simulink subsystem "Communication_Simulator"  (R2024a)
settings: Solver=VariableStepAuto  StartTime=0.0  StopTime=10.0  RelTol=1e-3
undefined symbols (not defined in the file): paramRFSatLink, QAM, rfSatSourceSamplesPerSymbol, rfSatSourceSampleTime
libraries: commrflib2 x24, dspsigops x12, commrfcorlib x8, commfilt2 x8, commdigbbndam3 x8, dspsolvers x8, simulink x8, commrandsrc3 x4, commsink2 x4, commdemoslib x4, impairlib x4, commsync2 x4
(part 3 of 3)

== system Communication_Simulator/TT&C Communication/Ground Segment/Downlink/Nonlinearity/Digital Pre-Distortion ==
  In1 : Inport
  In2 : Inport  Port=2
  Distortion compensation : Subsystem
  Parameter Estimation : Subsystem
  Out1 : Outport  VectorParamsAs1DForOutWhenUnconnected=off
  wires:
  In1/1 -> Distortion compensation/3(In), Parameter Estimation/1(DUT Input)
  Parameter Estimation/1(c) -> Distortion compensation/1(c)
  Parameter Estimation/2(d) -> Distortion compensation/2(d)
  Distortion compensation/1(Pre-distorted Signal) -> Out1/1
  In2/1 -> Parameter Estimation/2(DUT Output)

== system Communication_Simulator/TT&C Communication/Ground Segment/Ground Station/Nonlinearity1/Digital Pre-Distortion ==
  In1 : Inport
  In2 : Inport  Port=2
  Distortion compensation : Subsystem
  Parameter Estimation : Subsystem
  Out1 : Outport  VectorParamsAs1DForOutWhenUnconnected=off
  wires:
  In1/1 -> Distortion compensation/3(In), Parameter Estimation/1(DUT Input)
  Parameter Estimation/1(c) -> Distortion compensation/1(c)
  Parameter Estimation/2(d) -> Distortion compensation/2(d)
  Distortion compensation/1(Pre-distorted Signal) -> Out1/1
  In2/1 -> Parameter Estimation/2(DUT Output)

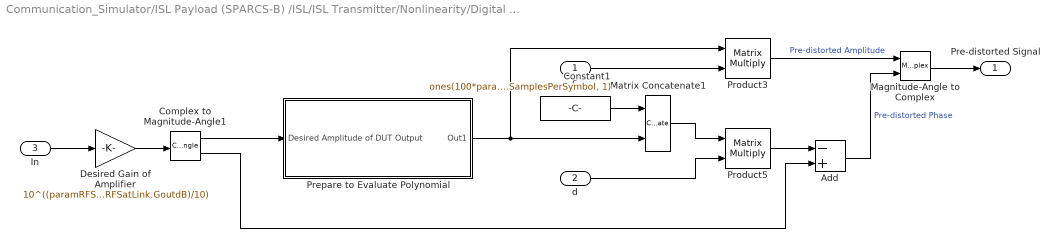
== system Communication_Simulator/ISL Payload (SPARCS-B) /ISL/ISL Transmitter/Nonlinearity/Digital Pre-Distortion/Distortion compensation ==
  c : Inport
  d : Inport  Port=2
  In : Inport  Port=3
  Add : Sum  Inputs=-+
  Complex to Magnitude-Angle1 : ComplexToMagnitudeAngle
  Constant1 : Constant  Value=ones(100*paramRFSatLink.SamplesPerSymbol, 1)
  Desired Gain of Amplifier : Gain  Gain=10^((paramRFSatLink.GindB + paramRFSatLink.GoutdB)/10)
  Magnitude-Angle to Complex : MagnitudeAngleToComplex
  Matrix Concatenate1 : Concatenate  Mode=Multidimensional array  ConcatenateDimension=2
  Prepare to Evaluate Polynomial : Subsystem
  Product3 : Product  Multiplication=Matrix(*)  RndMeth=Zero
  Product5 : Product  Multiplication=Matrix(*)  RndMeth=Zero
  Pre-distorted Signal : Outport  VectorParamsAs1DForOutWhenUnconnected=off
  wires:
  Desired Gain of Amplifier/1 -> Complex to Magnitude-Angle1/1
  c/1 -> Product3/2
  Add/1 -> Magnitude-Angle to Complex/2  "Pre-distorted Phase"
  Product5/1 -> Add/1
  Product3/1 -> Magnitude-Angle to Complex/1  "Pre-distorted Amplitude"
  d/1 -> Product5/2
  In/1 -> Desired Gain of Amplifier/1
  Magnitude-Angle to Complex/1 -> Pre-distorted Signal/1
  Complex to Magnitude-Angle1/2 -> Add/2
  Complex to Magnitude-Angle1/1 -> Prepare to Evaluate Polynomial/1(Desired Amplitude of DUT Output)
  Matrix Concatenate1/1 -> Product5/1
  Prepare to Evaluate Polynomial/1(Out1) -> Matrix Concatenate1/2, Product3/1
  Constant1/1 -> Matrix Concatenate1/1

== system Communication_Simulator/ISL Payload (SPARCS-B) /ISL/ISL Transmitter/Nonlinearity/Digital Pre-Distortion/Parameter Estimation ==
  DUT Input : Inport
  DUT Output : Inport  Port=2
  Complex to Magnitude-Angle : ComplexToMagnitudeAngle
  Complex to Magnitude-Angle1 : ComplexToMagnitudeAngle
  Polynomial Approximation : Subsystem
  c : Outport  VectorParamsAs1DForOutWhenUnconnected=off
  d : Outport  Port=2  VectorParamsAs1DForOutWhenUnconnected=off
  wires:
  DUT Input/1 -> Complex to Magnitude-Angle/1
  DUT Output/1 -> Complex to Magnitude-Angle1/1
  Complex to Magnitude-Angle1/1 -> Polynomial Approximation/3(Amplitude of DUT Output)
  Complex to Magnitude-Angle/2 -> Polynomial Approximation/2(Phase of DUT Input)
  Polynomial Approximation/1(Coef_c) -> c/1
  Polynomial Approximation/2(Coef_d) -> d/1
  Complex to Magnitude-Angle1/2 -> Polynomial Approximation/4(Phase of DUT Output)
  Complex to Magnitude-Angle/1 -> Polynomial Approximation/1(Amplitude of DUT Input)

== system Communication_Simulator/ISL Payload (SPARCS-B) /ISL/Other Satellite/Nonlinearity1/Digital Pre-Distortion/Distortion compensation ==
  c : Inport
  d : Inport  Port=2
  In : Inport  Port=3
  Add : Sum  Inputs=-+
  Complex to Magnitude-Angle1 : ComplexToMagnitudeAngle
  Constant1 : Constant  Value=ones(100*paramRFSatLink.SamplesPerSymbol, 1)
  Desired Gain of Amplifier : Gain  Gain=10^((paramRFSatLink.GindB + paramRFSatLink.GoutdB)/10)
  Magnitude-Angle to Complex : MagnitudeAngleToComplex
  Matrix Concatenate1 : Concatenate  Mode=Multidimensional array  ConcatenateDimension=2
  Prepare to Evaluate Polynomial : Subsystem
  Product3 : Product  Multiplication=Matrix(*)  RndMeth=Zero
  Product5 : Product  Multiplication=Matrix(*)  RndMeth=Zero
  Pre-distorted Signal : Outport  VectorParamsAs1DForOutWhenUnconnected=off
  wires:
  Desired Gain of Amplifier/1 -> Complex to Magnitude-Angle1/1
  c/1 -> Product3/2
  Add/1 -> Magnitude-Angle to Complex/2  "Pre-distorted Phase"
  Product5/1 -> Add/1
  Product3/1 -> Magnitude-Angle to Complex/1  "Pre-distorted Amplitude"
  d/1 -> Product5/2
  In/1 -> Desired Gain of Amplifier/1
  Magnitude-Angle to Complex/1 -> Pre-distorted Signal/1
  Complex to Magnitude-Angle1/2 -> Add/2
  Complex to Magnitude-Angle1/1 -> Prepare to Evaluate Polynomial/1(Desired Amplitude of DUT Output)
  Matrix Concatenate1/1 -> Product5/1
  Prepare to Evaluate Polynomial/1(Out1) -> Matrix Concatenate1/2, Product3/1
  Constant1/1 -> Matrix Concatenate1/1

== system Communication_Simulator/ISL Payload (SPARCS-B) /ISL/Other Satellite/Nonlinearity1/Digital Pre-Distortion/Parameter Estimation ==
  DUT Input : Inport
  DUT Output : Inport  Port=2
  Complex to Magnitude-Angle : ComplexToMagnitudeAngle
  Complex to Magnitude-Angle1 : ComplexToMagnitudeAngle
  Polynomial Approximation : Subsystem
  c : Outport  VectorParamsAs1DForOutWhenUnconnected=off
  d : Outport  Port=2  VectorParamsAs1DForOutWhenUnconnected=off
  wires:
  DUT Input/1 -> Complex to Magnitude-Angle/1
  DUT Output/1 -> Complex to Magnitude-Angle1/1
  Complex to Magnitude-Angle1/1 -> Polynomial Approximation/3(Amplitude of DUT Output)
  Complex to Magnitude-Angle/2 -> Polynomial Approximation/2(Phase of DUT Input)
  Polynomial Approximation/1(Coef_c) -> c/1
  Polynomial Approximation/2(Coef_d) -> d/1
  Complex to Magnitude-Angle1/2 -> Polynomial Approximation/4(Phase of DUT Output)
  Complex to Magnitude-Angle/1 -> Polynomial Approximation/1(Amplitude of DUT Input)

== system Communication_Simulator/TT&C Communication/Ground Segment/Downlink/Nonlinearity/Digital Pre-Distortion/Distortion compensation ==
  c : Inport
  d : Inport  Port=2
  In : Inport  Port=3
  Add : Sum  Inputs=-+
  Complex to Magnitude-Angle1 : ComplexToMagnitudeAngle
  Constant1 : Constant  Value=ones(100*paramRFSatLink.SamplesPerSymbol, 1)
  Desired Gain of Amplifier : Gain  Gain=10^((paramRFSatLink.GindB + paramRFSatLink.GoutdB)/10)
  Magnitude-Angle to Complex : MagnitudeAngleToComplex
  Matrix Concatenate1 : Concatenate  Mode=Multidimensional array  ConcatenateDimension=2
  Prepare to Evaluate Polynomial : Subsystem
  Product3 : Product  Multiplication=Matrix(*)  RndMeth=Zero
  Product5 : Product  Multiplication=Matrix(*)  RndMeth=Zero
  Pre-distorted Signal : Outport  VectorParamsAs1DForOutWhenUnconnected=off
  wires:
  Desired Gain of Amplifier/1 -> Complex to Magnitude-Angle1/1
  c/1 -> Product3/2
  Add/1 -> Magnitude-Angle to Complex/2  "Pre-distorted Phase"
  Product5/1 -> Add/1
  Product3/1 -> Magnitude-Angle to Complex/1  "Pre-distorted Amplitude"
  d/1 -> Product5/2
  In/1 -> Desired Gain of Amplifier/1
  Magnitude-Angle to Complex/1 -> Pre-distorted Signal/1
  Complex to Magnitude-Angle1/2 -> Add/2
  Complex to Magnitude-Angle1/1 -> Prepare to Evaluate Polynomial/1(Desired Amplitude of DUT Output)
  Matrix Concatenate1/1 -> Product5/1
  Prepare to Evaluate Polynomial/1(Out1) -> Matrix Concatenate1/2, Product3/1
  Constant1/1 -> Matrix Concatenate1/1

== system Communication_Simulator/TT&C Communication/Ground Segment/Downlink/Nonlinearity/Digital Pre-Distortion/Parameter Estimation ==
  DUT Input : Inport
  DUT Output : Inport  Port=2
  Complex to Magnitude-Angle : ComplexToMagnitudeAngle
  Complex to Magnitude-Angle1 : ComplexToMagnitudeAngle
  Polynomial Approximation : Subsystem
  c : Outport  VectorParamsAs1DForOutWhenUnconnected=off
  d : Outport  Port=2  VectorParamsAs1DForOutWhenUnconnected=off
  wires:
  DUT Input/1 -> Complex to Magnitude-Angle/1
  DUT Output/1 -> Complex to Magnitude-Angle1/1
  Complex to Magnitude-Angle1/1 -> Polynomial Approximation/3(Amplitude of DUT Output)
  Complex to Magnitude-Angle/2 -> Polynomial Approximation/2(Phase of DUT Input)
  Polynomial Approximation/1(Coef_c) -> c/1
  Polynomial Approximation/2(Coef_d) -> d/1
  Complex to Magnitude-Angle1/2 -> Polynomial Approximation/4(Phase of DUT Output)
  Complex to Magnitude-Angle/1 -> Polynomial Approximation/1(Amplitude of DUT Input)

== system Communication_Simulator/TT&C Communication/Ground Segment/Ground Station/Nonlinearity1/Digital Pre-Distortion/Distortion compensation ==
  c : Inport
  d : Inport  Port=2
  In : Inport  Port=3
  Add : Sum  Inputs=-+
  Complex to Magnitude-Angle1 : ComplexToMagnitudeAngle
  Constant1 : Constant  Value=ones(100*paramRFSatLink.SamplesPerSymbol, 1)
  Desired Gain of Amplifier : Gain  Gain=10^((paramRFSatLink.GindB + paramRFSatLink.GoutdB)/10)
  Magnitude-Angle to Complex : MagnitudeAngleToComplex
  Matrix Concatenate1 : Concatenate  Mode=Multidimensional array  ConcatenateDimension=2
  Prepare to Evaluate Polynomial : Subsystem
  Product3 : Product  Multiplication=Matrix(*)  RndMeth=Zero
  Product5 : Product  Multiplication=Matrix(*)  RndMeth=Zero
  Pre-distorted Signal : Outport  VectorParamsAs1DForOutWhenUnconnected=off
  wires:
  Desired Gain of Amplifier/1 -> Complex to Magnitude-Angle1/1
  c/1 -> Product3/2
  Add/1 -> Magnitude-Angle to Complex/2  "Pre-distorted Phase"
  Product5/1 -> Add/1
  Product3/1 -> Magnitude-Angle to Complex/1  "Pre-distorted Amplitude"
  d/1 -> Product5/2
  In/1 -> Desired Gain of Amplifier/1
  Magnitude-Angle to Complex/1 -> Pre-distorted Signal/1
  Complex to Magnitude-Angle1/2 -> Add/2
  Complex to Magnitude-Angle1/1 -> Prepare to Evaluate Polynomial/1(Desired Amplitude of DUT Output)
  Matrix Concatenate1/1 -> Product5/1
  Prepare to Evaluate Polynomial/1(Out1) -> Matrix Concatenate1/2, Product3/1
  Constant1/1 -> Matrix Concatenate1/1

== system Communication_Simulator/TT&C Communication/Ground Segment/Ground Station/Nonlinearity1/Digital Pre-Distortion/Parameter Estimation ==
  DUT Input : Inport
  DUT Output : Inport  Port=2
  Complex to Magnitude-Angle : ComplexToMagnitudeAngle
  Complex to Magnitude-Angle1 : ComplexToMagnitudeAngle
  Polynomial Approximation : Subsystem
  c : Outport  VectorParamsAs1DForOutWhenUnconnected=off
  d : Outport  Port=2  VectorParamsAs1DForOutWhenUnconnected=off
  wires:
  DUT Input/1 -> Complex to Magnitude-Angle/1
  DUT Output/1 -> Complex to Magnitude-Angle1/1
  Complex to Magnitude-Angle1/1 -> Polynomial Approximation/3(Amplitude of DUT Output)
  Complex to Magnitude-Angle/2 -> Polynomial Approximation/2(Phase of DUT Input)
  Polynomial Approximation/1(Coef_c) -> c/1
  Polynomial Approximation/2(Coef_d) -> d/1
  Complex to Magnitude-Angle1/2 -> Polynomial Approximation/4(Phase of DUT Output)
  Complex to Magnitude-Angle/1 -> Polynomial Approximation/1(Amplitude of DUT Input)

== system Communication_Simulator/ISL Payload (SPARCS-B) /ISL/ISL Transmitter/Nonlinearity/Digital Pre-Distortion/Distortion compensation/Prepare to Evaluate Polynomial ==
  Desired Amplitude of DUT Output : Inport
  Matrix Concatenate1 : Concatenate  NumInputs=5  Mode=Multidimensional array  ConcatenateDimension=2
  Product{6..9} (4 alike) : Product  RndMeth=Zero
  Out1 : Outport  VectorParamsAs1DForOutWhenUnconnected=off
  wires:
  Desired Amplitude of DUT Output/1 -> Product9/2, Product8/2, Product7/2, Product6/2, Product6/1, Matrix Concatenate1/1
  Product7/1 -> Product8/1, Matrix Concatenate1/3
  Product6/1 -> Product7/1, Matrix Concatenate1/2
  Product8/1 -> Product9/1, Matrix Concatenate1/4
  Product9/1 -> Matrix Concatenate1/5
  Matrix Concatenate1/1 -> Out1/1

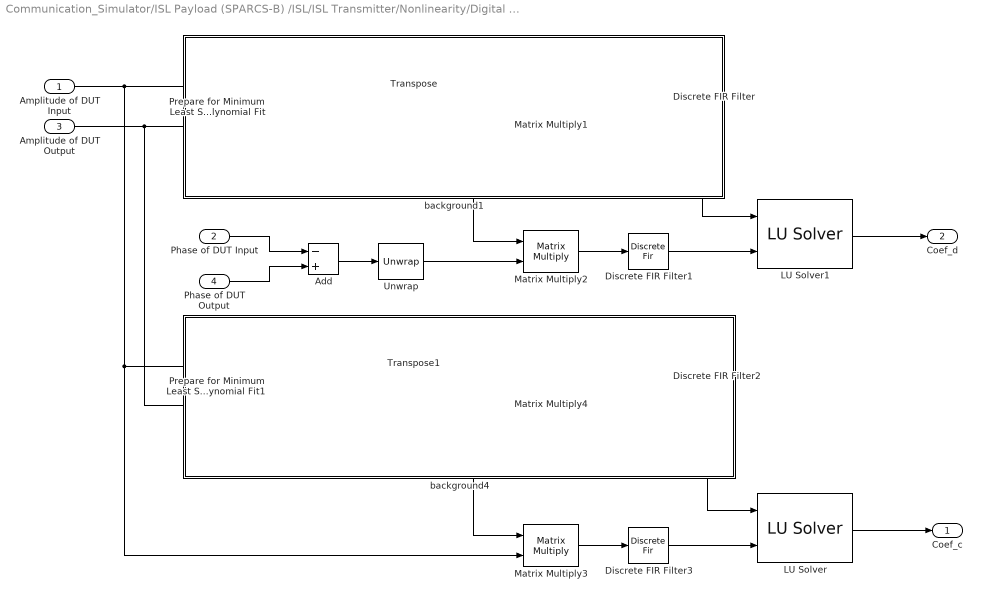
== system Communication_Simulator/ISL Payload (SPARCS-B) /ISL/ISL Transmitter/Nonlinearity/Digital Pre-Distortion/Parameter Estimation/Polynomial Approximation ==
  Amplitude of DUT Input : Inport
  Phase of DUT Input : Inport  Port=2
  Amplitude of DUT Output : Inport  Port=3
  Phase of DUT Output : Inport  Port=4
  Add : Sum  Inputs=-+
  Discrete FIR Filter{,1..3} (4 alike) : DiscreteFir  Coefficients=ones(1,50)  AccumDataTypeStr=Inherit: Same as product output
  LU Solver : dspsolvers/LU Solver
  LU Solver1 : dspsolvers/LU Solver
  Matrix Multiply{1..4} (4 alike) : Product  Multiplication=Matrix(*)
  Prepare for Minimum Least Square Error Polynomial Fit : Subsystem
  Prepare for Minimum Least Square Error Polynomial Fit1 : Subsystem
  Transpose : Math  Operator=transpose  SignedPower=on
  Transpose1 : Math  Operator=transpose  SignedPower=on
  Unwrap : dspsigops/Unwrap  tol=pi  InputProcessing=Columns as channels (frame based)  running=off
  background1 : Subsystem
      mask Display: disp('')
  background4 : Subsystem
      mask Display: disp('')
  Coef_c : Outport  VectorParamsAs1DForOutWhenUnconnected=off
  Coef_d : Outport  Port=2  VectorParamsAs1DForOutWhenUnconnected=off
  wires:
  Discrete FIR Filter2/1 -> LU Solver/1
  Transpose1/1 -> Matrix Multiply3/1, Matrix Multiply4/1
  Matrix Multiply4/1 -> Discrete FIR Filter2/1
  Prepare for Minimum Least Square Error Polynomial Fit1/1(Out1) -> Matrix Multiply4/2, Transpose1/1
  Phase of DUT Input/1 -> Add/1
  Add/1 -> Unwrap/1
  Amplitude of DUT Input/1 -> Prepare for Minimum Least Square Error Polynomial Fit/1(In1), Prepare for Minimum Least Square Error Polynomial Fit1/1(In1), Matrix Multiply3/2
  Matrix Multiply1/1 -> Discrete FIR Filter/1
  Matrix Multiply3/1 -> Discrete FIR Filter3/1
  Prepare for Minimum Least Square Error Polynomial Fit/1(Out1) -> Matrix Multiply1/2, Transpose/1
  Unwrap/1 -> Matrix Multiply2/2
  Matrix Multiply2/1 -> Discrete FIR Filter1/1
  Amplitude of DUT Output/1 -> Prepare for Minimum Least Square Error Polynomial Fit1/2(In2), Prepare for Minimum Least Square Error Polynomial Fit/2(In2)
  Discrete FIR Filter1/1 -> LU Solver1/2
  Discrete FIR Filter/1 -> LU Solver1/1
  Discrete FIR Filter3/1 -> LU Solver/2
  Phase of DUT Output/1 -> Add/2
  LU Solver1/1 -> Coef_d/1
  LU Solver/1 -> Coef_c/1
  Transpose/1 -> Matrix Multiply1/1, Matrix Multiply2/1

== system Communication_Simulator/ISL Payload (SPARCS-B) /ISL/Other Satellite/Nonlinearity1/Digital Pre-Distortion/Distortion compensation/Prepare to Evaluate Polynomial ==
  Desired Amplitude of DUT Output : Inport
  Matrix Concatenate1 : Concatenate  NumInputs=5  Mode=Multidimensional array  ConcatenateDimension=2
  Product{6..9} (4 alike) : Product  RndMeth=Zero
  Out1 : Outport  VectorParamsAs1DForOutWhenUnconnected=off
  wires:
  Desired Amplitude of DUT Output/1 -> Product9/2, Product8/2, Product7/2, Product6/2, Product6/1, Matrix Concatenate1/1
  Product7/1 -> Product8/1, Matrix Concatenate1/3
  Product6/1 -> Product7/1, Matrix Concatenate1/2
  Product8/1 -> Product9/1, Matrix Concatenate1/4
  Product9/1 -> Matrix Concatenate1/5
  Matrix Concatenate1/1 -> Out1/1

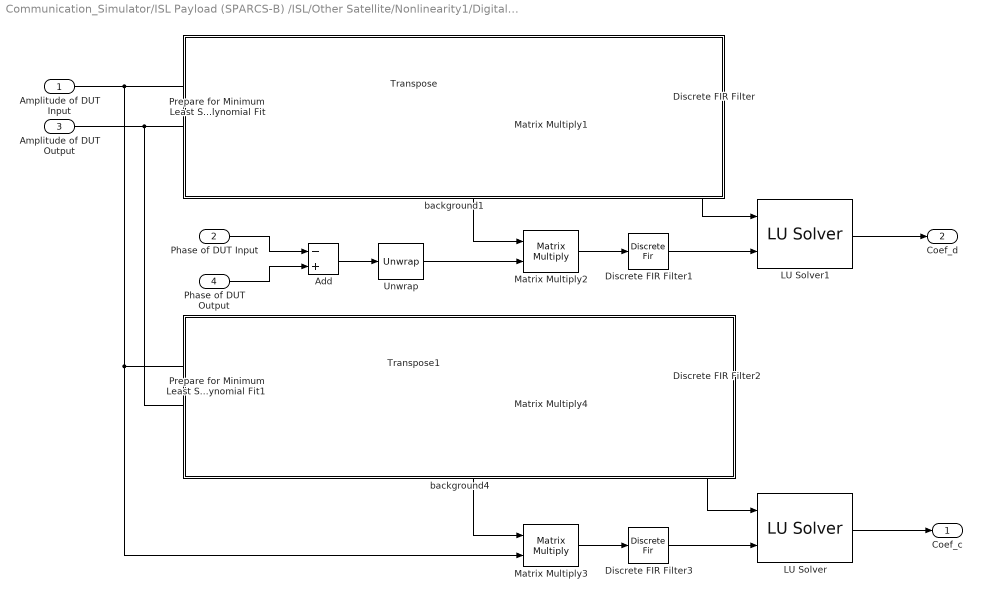
== system Communication_Simulator/ISL Payload (SPARCS-B) /ISL/Other Satellite/Nonlinearity1/Digital Pre-Distortion/Parameter Estimation/Polynomial Approximation ==
  Amplitude of DUT Input : Inport
  Phase of DUT Input : Inport  Port=2
  Amplitude of DUT Output : Inport  Port=3
  Phase of DUT Output : Inport  Port=4
  Add : Sum  Inputs=-+
  Discrete FIR Filter{,1..3} (4 alike) : DiscreteFir  Coefficients=ones(1,50)  AccumDataTypeStr=Inherit: Same as product output
  LU Solver : dspsolvers/LU Solver
  LU Solver1 : dspsolvers/LU Solver
  Matrix Multiply{1..4} (4 alike) : Product  Multiplication=Matrix(*)
  Prepare for Minimum Least Square Error Polynomial Fit : Subsystem
  Prepare for Minimum Least Square Error Polynomial Fit1 : Subsystem
  Transpose : Math  Operator=transpose  SignedPower=on
  Transpose1 : Math  Operator=transpose  SignedPower=on
  Unwrap : dspsigops/Unwrap  tol=pi  InputProcessing=Columns as channels (frame based)  running=off
  background1 : Subsystem
      mask Display: disp('')
  background4 : Subsystem
      mask Display: disp('')
  Coef_c : Outport  VectorParamsAs1DForOutWhenUnconnected=off
  Coef_d : Outport  Port=2  VectorParamsAs1DForOutWhenUnconnected=off
  wires:
  Discrete FIR Filter2/1 -> LU Solver/1
  Transpose1/1 -> Matrix Multiply3/1, Matrix Multiply4/1
  Matrix Multiply4/1 -> Discrete FIR Filter2/1
  Prepare for Minimum Least Square Error Polynomial Fit1/1(Out1) -> Matrix Multiply4/2, Transpose1/1
  Phase of DUT Input/1 -> Add/1
  Add/1 -> Unwrap/1
  Amplitude of DUT Input/1 -> Prepare for Minimum Least Square Error Polynomial Fit/1(In1), Prepare for Minimum Least Square Error Polynomial Fit1/1(In1), Matrix Multiply3/2
  Matrix Multiply1/1 -> Discrete FIR Filter/1
  Matrix Multiply3/1 -> Discrete FIR Filter3/1
  Prepare for Minimum Least Square Error Polynomial Fit/1(Out1) -> Matrix Multiply1/2, Transpose/1
  Unwrap/1 -> Matrix Multiply2/2
  Matrix Multiply2/1 -> Discrete FIR Filter1/1
  Amplitude of DUT Output/1 -> Prepare for Minimum Least Square Error Polynomial Fit1/2(In2), Prepare for Minimum Least Square Error Polynomial Fit/2(In2)
  Discrete FIR Filter1/1 -> LU Solver1/2
  Discrete FIR Filter/1 -> LU Solver1/1
  Discrete FIR Filter3/1 -> LU Solver/2
  Phase of DUT Output/1 -> Add/2
  LU Solver1/1 -> Coef_d/1
  LU Solver/1 -> Coef_c/1
  Transpose/1 -> Matrix Multiply1/1, Matrix Multiply2/1

== system Communication_Simulator/TT&C Communication/Ground Segment/Downlink/Nonlinearity/Digital Pre-Distortion/Distortion compensation/Prepare to Evaluate Polynomial ==
  Desired Amplitude of DUT Output : Inport
  Matrix Concatenate1 : Concatenate  NumInputs=5  Mode=Multidimensional array  ConcatenateDimension=2
  Product{6..9} (4 alike) : Product  RndMeth=Zero
  Out1 : Outport  VectorParamsAs1DForOutWhenUnconnected=off
  wires:
  Desired Amplitude of DUT Output/1 -> Product9/2, Product8/2, Product7/2, Product6/2, Product6/1, Matrix Concatenate1/1
  Product7/1 -> Product8/1, Matrix Concatenate1/3
  Product6/1 -> Product7/1, Matrix Concatenate1/2
  Product8/1 -> Product9/1, Matrix Concatenate1/4
  Product9/1 -> Matrix Concatenate1/5
  Matrix Concatenate1/1 -> Out1/1

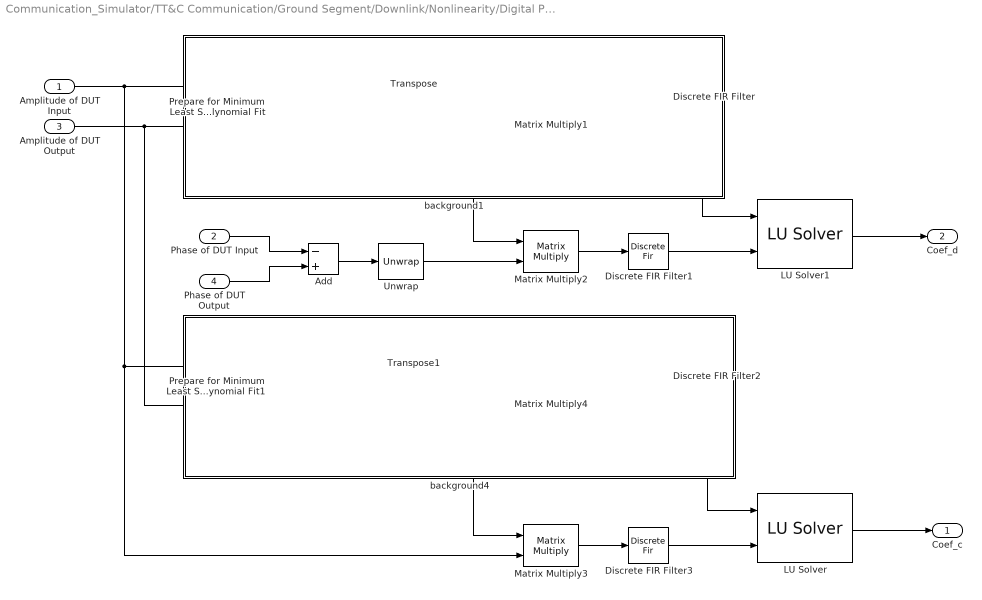
== system Communication_Simulator/TT&C Communication/Ground Segment/Downlink/Nonlinearity/Digital Pre-Distortion/Parameter Estimation/Polynomial Approximation ==
  Amplitude of DUT Input : Inport
  Phase of DUT Input : Inport  Port=2
  Amplitude of DUT Output : Inport  Port=3
  Phase of DUT Output : Inport  Port=4
  Add : Sum  Inputs=-+
  Discrete FIR Filter{,1..3} (4 alike) : DiscreteFir  Coefficients=ones(1,50)  AccumDataTypeStr=Inherit: Same as product output
  LU Solver : dspsolvers/LU Solver
  LU Solver1 : dspsolvers/LU Solver
  Matrix Multiply{1..4} (4 alike) : Product  Multiplication=Matrix(*)
  Prepare for Minimum Least Square Error Polynomial Fit : Subsystem
  Prepare for Minimum Least Square Error Polynomial Fit1 : Subsystem
  Transpose : Math  Operator=transpose  SignedPower=on
  Transpose1 : Math  Operator=transpose  SignedPower=on
  Unwrap : dspsigops/Unwrap  tol=pi  InputProcessing=Columns as channels (frame based)  running=off
  background1 : Subsystem
      mask Display: disp('')
  background4 : Subsystem
      mask Display: disp('')
  Coef_c : Outport  VectorParamsAs1DForOutWhenUnconnected=off
  Coef_d : Outport  Port=2  VectorParamsAs1DForOutWhenUnconnected=off
  wires:
  Discrete FIR Filter2/1 -> LU Solver/1
  Transpose1/1 -> Matrix Multiply3/1, Matrix Multiply4/1
  Matrix Multiply4/1 -> Discrete FIR Filter2/1
  Prepare for Minimum Least Square Error Polynomial Fit1/1(Out1) -> Matrix Multiply4/2, Transpose1/1
  Phase of DUT Input/1 -> Add/1
  Add/1 -> Unwrap/1
  Amplitude of DUT Input/1 -> Prepare for Minimum Least Square Error Polynomial Fit/1(In1), Prepare for Minimum Least Square Error Polynomial Fit1/1(In1), Matrix Multiply3/2
  Matrix Multiply1/1 -> Discrete FIR Filter/1
  Matrix Multiply3/1 -> Discrete FIR Filter3/1
  Prepare for Minimum Least Square Error Polynomial Fit/1(Out1) -> Matrix Multiply1/2, Transpose/1
  Unwrap/1 -> Matrix Multiply2/2
  Matrix Multiply2/1 -> Discrete FIR Filter1/1
  Amplitude of DUT Output/1 -> Prepare for Minimum Least Square Error Polynomial Fit1/2(In2), Prepare for Minimum Least Square Error Polynomial Fit/2(In2)
  Discrete FIR Filter1/1 -> LU Solver1/2
  Discrete FIR Filter/1 -> LU Solver1/1
  Discrete FIR Filter3/1 -> LU Solver/2
  Phase of DUT Output/1 -> Add/2
  LU Solver1/1 -> Coef_d/1
  LU Solver/1 -> Coef_c/1
  Transpose/1 -> Matrix Multiply1/1, Matrix Multiply2/1

== system Communication_Simulator/TT&C Communication/Ground Segment/Ground Station/Nonlinearity1/Digital Pre-Distortion/Distortion compensation/Prepare to Evaluate Polynomial ==
  Desired Amplitude of DUT Output : Inport
  Matrix Concatenate1 : Concatenate  NumInputs=5  Mode=Multidimensional array  ConcatenateDimension=2
  Product{6..9} (4 alike) : Product  RndMeth=Zero
  Out1 : Outport  VectorParamsAs1DForOutWhenUnconnected=off
  wires:
  Desired Amplitude of DUT Output/1 -> Product9/2, Product8/2, Product7/2, Product6/2, Product6/1, Matrix Concatenate1/1
  Product7/1 -> Product8/1, Matrix Concatenate1/3
  Product6/1 -> Product7/1, Matrix Concatenate1/2
  Product8/1 -> Product9/1, Matrix Concatenate1/4
  Product9/1 -> Matrix Concatenate1/5
  Matrix Concatenate1/1 -> Out1/1

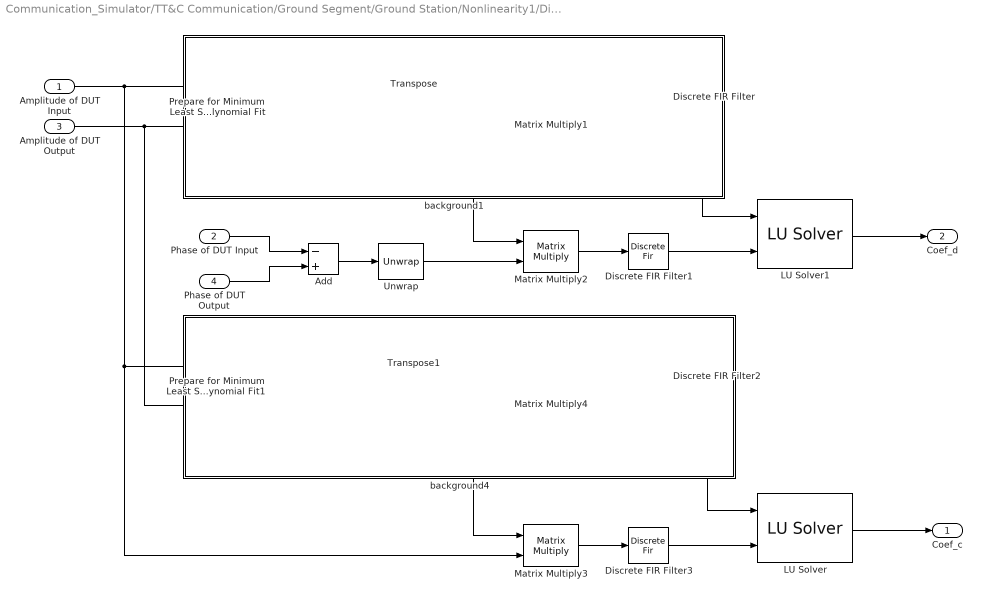
== system Communication_Simulator/TT&C Communication/Ground Segment/Ground Station/Nonlinearity1/Digital Pre-Distortion/Parameter Estimation/Polynomial Approximation ==
  Amplitude of DUT Input : Inport
  Phase of DUT Input : Inport  Port=2
  Amplitude of DUT Output : Inport  Port=3
  Phase of DUT Output : Inport  Port=4
  Add : Sum  Inputs=-+
  Discrete FIR Filter{,1..3} (4 alike) : DiscreteFir  Coefficients=ones(1,50)  AccumDataTypeStr=Inherit: Same as product output
  LU Solver : dspsolvers/LU Solver
  LU Solver1 : dspsolvers/LU Solver
  Matrix Multiply{1..4} (4 alike) : Product  Multiplication=Matrix(*)
  Prepare for Minimum Least Square Error Polynomial Fit : Subsystem
  Prepare for Minimum Least Square Error Polynomial Fit1 : Subsystem
  Transpose : Math  Operator=transpose  SignedPower=on
  Transpose1 : Math  Operator=transpose  SignedPower=on
  Unwrap : dspsigops/Unwrap  tol=pi  InputProcessing=Columns as channels (frame based)  running=off
  background1 : Subsystem
      mask Display: disp('')
  background4 : Subsystem
      mask Display: disp('')
  Coef_c : Outport  VectorParamsAs1DForOutWhenUnconnected=off
  Coef_d : Outport  Port=2  VectorParamsAs1DForOutWhenUnconnected=off
  wires:
  Discrete FIR Filter2/1 -> LU Solver/1
  Transpose1/1 -> Matrix Multiply3/1, Matrix Multiply4/1
  Matrix Multiply4/1 -> Discrete FIR Filter2/1
  Prepare for Minimum Least Square Error Polynomial Fit1/1(Out1) -> Matrix Multiply4/2, Transpose1/1
  Phase of DUT Input/1 -> Add/1
  Add/1 -> Unwrap/1
  Amplitude of DUT Input/1 -> Prepare for Minimum Least Square Error Polynomial Fit/1(In1), Prepare for Minimum Least Square Error Polynomial Fit1/1(In1), Matrix Multiply3/2
  Matrix Multiply1/1 -> Discrete FIR Filter/1
  Matrix Multiply3/1 -> Discrete FIR Filter3/1
  Prepare for Minimum Least Square Error Polynomial Fit/1(Out1) -> Matrix Multiply1/2, Transpose/1
  Unwrap/1 -> Matrix Multiply2/2
  Matrix Multiply2/1 -> Discrete FIR Filter1/1
  Amplitude of DUT Output/1 -> Prepare for Minimum Least Square Error Polynomial Fit1/2(In2), Prepare for Minimum Least Square Error Polynomial Fit/2(In2)
  Discrete FIR Filter1/1 -> LU Solver1/2
  Discrete FIR Filter/1 -> LU Solver1/1
  Discrete FIR Filter3/1 -> LU Solver/2
  Phase of DUT Output/1 -> Add/2
  LU Solver1/1 -> Coef_d/1
  LU Solver/1 -> Coef_c/1
  Transpose/1 -> Matrix Multiply1/1, Matrix Multiply2/1

== system Communication_Simulator/ISL Payload (SPARCS-B) /ISL/ISL Transmitter/Nonlinearity/Digital Pre-Distortion/Parameter Estimation/Polynomial Approximation/Prepare for Minimum Least Square Error Polynomial Fit ==
  In1 : Inport
  In2 : Inport  Port=2
  Compare To Constant : simulink/Logic and Bit Operations/Compare To Constant  relop=>=  const=1e-3  OutDataTypeStr=uint8  ZeroCross=off
  Data Type Conversion : DataTypeConversion  OutDataTypeStr=double  SaturateOnIntegerOverflow=off  RndMeth=Floor
  Matrix Concatenate1 : Concatenate  NumInputs=6  Mode=Multidimensional array  ConcatenateDimension=2
  Product{,2..5} (5 alike) : Product  RndMeth=Zero
  Out1 : Outport  VectorParamsAs1DForOutWhenUnconnected=off
  wires:
  Compare To Constant/1 -> Product4/1, Data Type Conversion/1
  In2/1 -> Product4/2
  Product3/1 -> Product5/1, Matrix Concatenate1/5
  Product2/1 -> Product3/1, Matrix Concatenate1/4
  Product/1 -> Product2/1, Matrix Concatenate1/3
  Product4/1 -> Matrix Concatenate1/2, Product5/2, Product3/2, Product2/2, Product/2, Product/1
  Product5/1 -> Matrix Concatenate1/6
  Matrix Concatenate1/1 -> Out1/1
  In1/1 -> Compare To Constant/1
  Data Type Conversion/1 -> Matrix Concatenate1/1

== system Communication_Simulator/ISL Payload (SPARCS-B) /ISL/ISL Transmitter/Nonlinearity/Digital Pre-Distortion/Parameter Estimation/Polynomial Approximation/Prepare for Minimum Least Square Error Polynomial Fit1 ==
  In1 : Inport
  In2 : Inport  Port=2
  Compare To Constant : simulink/Logic and Bit Operations/Compare To Constant  relop=>=  const=1e-3  OutDataTypeStr=uint8  ZeroCross=off
  Data Type Conversion : DataTypeConversion  OutDataTypeStr=double  SaturateOnIntegerOverflow=off  RndMeth=Floor
  Matrix Concatenate1 : Concatenate  NumInputs=5  Mode=Multidimensional array  ConcatenateDimension=2
  Product{,2..5} (5 alike) : Product  RndMeth=Zero
  Out1 : Outport  VectorParamsAs1DForOutWhenUnconnected=off
  wires:
  Compare To Constant/1 -> Product4/1
  Data Type Conversion/1 -> Matrix Concatenate1/1
  In2/1 -> Product4/2
  Product/1 -> Matrix Concatenate1/2, Product2/1
  Product4/1 -> Data Type Conversion/1, Product2/2, Product3/2, Product5/2, Product/2, Product/1
  Product5/1 -> Matrix Concatenate1/5
  Product3/1 -> Matrix Concatenate1/4, Product5/1
  Product2/1 -> Matrix Concatenate1/3, Product3/1
  Matrix Concatenate1/1 -> Out1/1
  In1/1 -> Compare To Constant/1

== system Communication_Simulator/ISL Payload (SPARCS-B) /ISL/ISL Transmitter/Nonlinearity/Digital Pre-Distortion/Parameter Estimation/Polynomial Approximation/background1 ==

== system Communication_Simulator/ISL Payload (SPARCS-B) /ISL/ISL Transmitter/Nonlinearity/Digital Pre-Distortion/Parameter Estimation/Polynomial Approximation/background4 ==

== system Communication_Simulator/ISL Payload (SPARCS-B) /ISL/Other Satellite/Nonlinearity1/Digital Pre-Distortion/Parameter Estimation/Polynomial Approximation/Prepare for Minimum Least Square Error Polynomial Fit ==
  In1 : Inport
  In2 : Inport  Port=2
  Compare To Constant : simulink/Logic and Bit Operations/Compare To Constant  relop=>=  const=1e-3  OutDataTypeStr=uint8  ZeroCross=off
  Data Type Conversion : DataTypeConversion  OutDataTypeStr=double  SaturateOnIntegerOverflow=off  RndMeth=Floor
  Matrix Concatenate1 : Concatenate  NumInputs=6  Mode=Multidimensional array  ConcatenateDimension=2
  Product{,2..5} (5 alike) : Product  RndMeth=Zero
  Out1 : Outport  VectorParamsAs1DForOutWhenUnconnected=off
  wires:
  Compare To Constant/1 -> Product4/1, Data Type Conversion/1
  In2/1 -> Product4/2
  Product3/1 -> Product5/1, Matrix Concatenate1/5
  Product2/1 -> Product3/1, Matrix Concatenate1/4
  Product/1 -> Product2/1, Matrix Concatenate1/3
  Product4/1 -> Matrix Concatenate1/2, Product5/2, Product3/2, Product2/2, Product/2, Product/1
  Product5/1 -> Matrix Concatenate1/6
  Matrix Concatenate1/1 -> Out1/1
  In1/1 -> Compare To Constant/1
  Data Type Conversion/1 -> Matrix Concatenate1/1

== system Communication_Simulator/ISL Payload (SPARCS-B) /ISL/Other Satellite/Nonlinearity1/Digital Pre-Distortion/Parameter Estimation/Polynomial Approximation/Prepare for Minimum Least Square Error Polynomial Fit1 ==
  In1 : Inport
  In2 : Inport  Port=2
  Compare To Constant : simulink/Logic and Bit Operations/Compare To Constant  relop=>=  const=1e-3  OutDataTypeStr=uint8  ZeroCross=off
  Data Type Conversion : DataTypeConversion  OutDataTypeStr=double  SaturateOnIntegerOverflow=off  RndMeth=Floor
  Matrix Concatenate1 : Concatenate  NumInputs=5  Mode=Multidimensional array  ConcatenateDimension=2
  Product{,2..5} (5 alike) : Product  RndMeth=Zero
  Out1 : Outport  VectorParamsAs1DForOutWhenUnconnected=off
  wires:
  Compare To Constant/1 -> Product4/1
  Data Type Conversion/1 -> Matrix Concatenate1/1
  In2/1 -> Product4/2
  Product/1 -> Matrix Concatenate1/2, Product2/1
  Product4/1 -> Data Type Conversion/1, Product2/2, Product3/2, Product5/2, Product/2, Product/1
  Product5/1 -> Matrix Concatenate1/5
  Product3/1 -> Matrix Concatenate1/4, Product5/1
  Product2/1 -> Matrix Concatenate1/3, Product3/1
  Matrix Concatenate1/1 -> Out1/1
  In1/1 -> Compare To Constant/1

== system Communication_Simulator/ISL Payload (SPARCS-B) /ISL/Other Satellite/Nonlinearity1/Digital Pre-Distortion/Parameter Estimation/Polynomial Approximation/background1 ==

== system Communication_Simulator/ISL Payload (SPARCS-B) /ISL/Other Satellite/Nonlinearity1/Digital Pre-Distortion/Parameter Estimation/Polynomial Approximation/background4 ==

== system Communication_Simulator/TT&C Communication/Ground Segment/Downlink/Nonlinearity/Digital Pre-Distortion/Parameter Estimation/Polynomial Approximation/Prepare for Minimum Least Square Error Polynomial Fit ==
  In1 : Inport
  In2 : Inport  Port=2
  Compare To Constant : simulink/Logic and Bit Operations/Compare To Constant  relop=>=  const=1e-3  OutDataTypeStr=uint8  ZeroCross=off
  Data Type Conversion : DataTypeConversion  OutDataTypeStr=double  SaturateOnIntegerOverflow=off  RndMeth=Floor
  Matrix Concatenate1 : Concatenate  NumInputs=6  Mode=Multidimensional array  ConcatenateDimension=2
  Product{,2..5} (5 alike) : Product  RndMeth=Zero
  Out1 : Outport  VectorParamsAs1DForOutWhenUnconnected=off
  wires:
  Compare To Constant/1 -> Product4/1, Data Type Conversion/1
  In2/1 -> Product4/2
  Product3/1 -> Product5/1, Matrix Concatenate1/5
  Product2/1 -> Product3/1, Matrix Concatenate1/4
  Product/1 -> Product2/1, Matrix Concatenate1/3
  Product4/1 -> Matrix Concatenate1/2, Product5/2, Product3/2, Product2/2, Product/2, Product/1
  Product5/1 -> Matrix Concatenate1/6
  Matrix Concatenate1/1 -> Out1/1
  In1/1 -> Compare To Constant/1
  Data Type Conversion/1 -> Matrix Concatenate1/1

== system Communication_Simulator/TT&C Communication/Ground Segment/Downlink/Nonlinearity/Digital Pre-Distortion/Parameter Estimation/Polynomial Approximation/Prepare for Minimum Least Square Error Polynomial Fit1 ==
  In1 : Inport
  In2 : Inport  Port=2
  Compare To Constant : simulink/Logic and Bit Operations/Compare To Constant  relop=>=  const=1e-3  OutDataTypeStr=uint8  ZeroCross=off
  Data Type Conversion : DataTypeConversion  OutDataTypeStr=double  SaturateOnIntegerOverflow=off  RndMeth=Floor
  Matrix Concatenate1 : Concatenate  NumInputs=5  Mode=Multidimensional array  ConcatenateDimension=2
  Product{,2..5} (5 alike) : Product  RndMeth=Zero
  Out1 : Outport  VectorParamsAs1DForOutWhenUnconnected=off
  wires:
  Compare To Constant/1 -> Product4/1
  Data Type Conversion/1 -> Matrix Concatenate1/1
  In2/1 -> Product4/2
  Product/1 -> Matrix Concatenate1/2, Product2/1
  Product4/1 -> Data Type Conversion/1, Product2/2, Product3/2, Product5/2, Product/2, Product/1
  Product5/1 -> Matrix Concatenate1/5
  Product3/1 -> Matrix Concatenate1/4, Product5/1
  Product2/1 -> Matrix Concatenate1/3, Product3/1
  Matrix Concatenate1/1 -> Out1/1
  In1/1 -> Compare To Constant/1

== system Communication_Simulator/TT&C Communication/Ground Segment/Downlink/Nonlinearity/Digital Pre-Distortion/Parameter Estimation/Polynomial Approximation/background1 ==

== system Communication_Simulator/TT&C Communication/Ground Segment/Downlink/Nonlinearity/Digital Pre-Distortion/Parameter Estimation/Polynomial Approximation/background4 ==

== system Communication_Simulator/TT&C Communication/Ground Segment/Ground Station/Nonlinearity1/Digital Pre-Distortion/Parameter Estimation/Polynomial Approximation/Prepare for Minimum Least Square Error Polynomial Fit ==
  In1 : Inport
  In2 : Inport  Port=2
  Compare To Constant : simulink/Logic and Bit Operations/Compare To Constant  relop=>=  const=1e-3  OutDataTypeStr=uint8  ZeroCross=off
  Data Type Conversion : DataTypeConversion  OutDataTypeStr=double  SaturateOnIntegerOverflow=off  RndMeth=Floor
  Matrix Concatenate1 : Concatenate  NumInputs=6  Mode=Multidimensional array  ConcatenateDimension=2
  Product{,2..5} (5 alike) : Product  RndMeth=Zero
  Out1 : Outport  VectorParamsAs1DForOutWhenUnconnected=off
  wires:
  Compare To Constant/1 -> Product4/1, Data Type Conversion/1
  In2/1 -> Product4/2
  Product3/1 -> Product5/1, Matrix Concatenate1/5
  Product2/1 -> Product3/1, Matrix Concatenate1/4
  Product/1 -> Product2/1, Matrix Concatenate1/3
  Product4/1 -> Matrix Concatenate1/2, Product5/2, Product3/2, Product2/2, Product/2, Product/1
  Product5/1 -> Matrix Concatenate1/6
  Matrix Concatenate1/1 -> Out1/1
  In1/1 -> Compare To Constant/1
  Data Type Conversion/1 -> Matrix Concatenate1/1

== system Communication_Simulator/TT&C Communication/Ground Segment/Ground Station/Nonlinearity1/Digital Pre-Distortion/Parameter Estimation/Polynomial Approximation/Prepare for Minimum Least Square Error Polynomial Fit1 ==
  In1 : Inport
  In2 : Inport  Port=2
  Compare To Constant : simulink/Logic and Bit Operations/Compare To Constant  relop=>=  const=1e-3  OutDataTypeStr=uint8  ZeroCross=off
  Data Type Conversion : DataTypeConversion  OutDataTypeStr=double  SaturateOnIntegerOverflow=off  RndMeth=Floor
  Matrix Concatenate1 : Concatenate  NumInputs=5  Mode=Multidimensional array  ConcatenateDimension=2
  Product{,2..5} (5 alike) : Product  RndMeth=Zero
  Out1 : Outport  VectorParamsAs1DForOutWhenUnconnected=off
  wires:
  Compare To Constant/1 -> Product4/1
  Data Type Conversion/1 -> Matrix Concatenate1/1
  In2/1 -> Product4/2
  Product/1 -> Matrix Concatenate1/2, Product2/1
  Product4/1 -> Data Type Conversion/1, Product2/2, Product3/2, Product5/2, Product/2, Product/1
  Product5/1 -> Matrix Concatenate1/5
  Product3/1 -> Matrix Concatenate1/4, Product5/1
  Product2/1 -> Matrix Concatenate1/3, Product3/1
  Matrix Concatenate1/1 -> Out1/1
  In1/1 -> Compare To Constant/1

== system Communication_Simulator/TT&C Communication/Ground Segment/Ground Station/Nonlinearity1/Digital Pre-Distortion/Parameter Estimation/Polynomial Approximation/background1 ==

== system Communication_Simulator/TT&C Communication/Ground Segment/Ground Station/Nonlinearity1/Digital Pre-Distortion/Parameter Estimation/Polynomial Approximation/background4 ==
